simulink model "pole_placement_oldversion"  (R2022a)
settings: Solver=FixedStepAuto  StartTime=0.0  StopTime=10  FixedStep=0.001  RelTol=1e-3
values from neighbouring files (symbols this model uses):
  A = [0 1.51506314161 0 -114.917471751 0 1 -372.885867158 0 797.381461885 0 0 0.563745877458 ... (25 elements, 5x5)]    [System.mat]    (also in linearize_operating_point.m = double(A))
  B = [0 0 0 0 863.333333333]    [System.mat]    (also in linearize_operating_point.m = double(B))
  C = [1  0  0  0  0; 0  0  1  0  0]    [System.mat]    (also in linearize_operating_point.m = [1 0 0 0 0)
  D = [0 0]    [System.mat]    (also in linearize_operating_point.m = zeros(2,1))
  K = K1    [controller.m]
  Ke = place(A_, B_, 2*J)'    [controller.m]
  T_0 = x_op(5)    [controller.m]    (also in run_compare_lin_non_lin.m)
  theta_1_0 = x_op(1)    [controller.m]    (also in run_compare_lin_non_lin.m)
  theta_2_0 = x_op(3)    [controller.m]    (also in run_compare_lin_non_lin.m)
  theta_d_1_0 = x_op(2)    [controller.m]    (also in run_compare_lin_non_lin.m)
  theta_d_2_0 = x_op(4)    [controller.m]    (also in run_compare_lin_non_lin.m)
  x_op = [3.14159265359 0 0 0 0]    [System.mat]    (also in linearize_operating_point.m = [init_theta_1; 0; init_theta_2; 0; 0])
  x_op_relative = [0; 0; 0; 0; 0]    [controller.m]
libraries: slpidlib x4
(part 1 of 3)
settings Model: Creator=annel  LastModifiedBy=97083
settings ModelReferenceCC: EnableRefExpFcnMdlSchedulingChecks=off
settings RTWCC: Description=Generic Real-Time Target

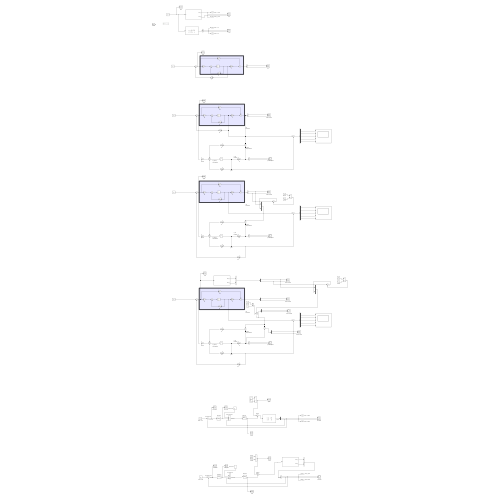
[thumbnail: Simulink's stored preview of the top-level diagram]
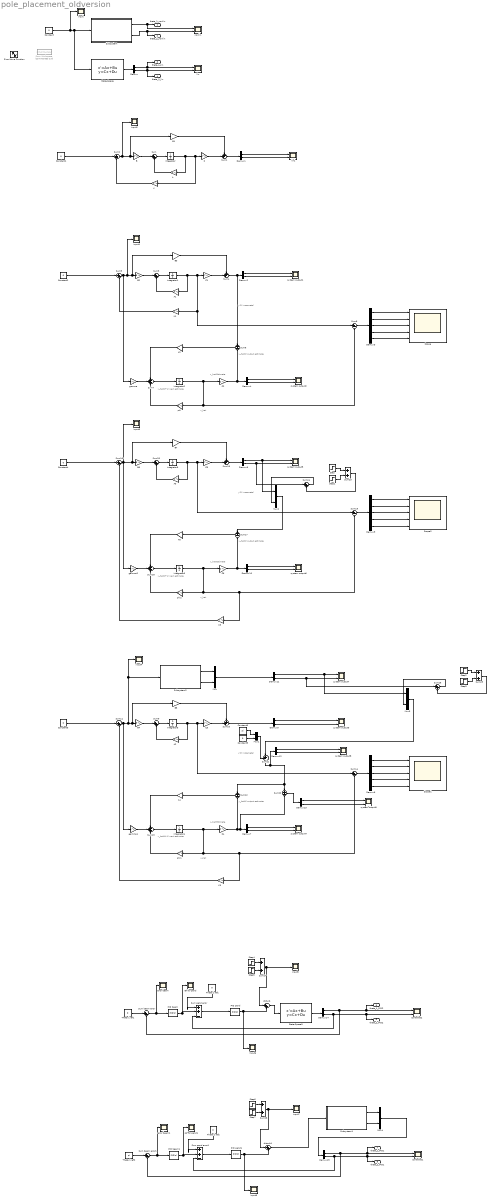
== system pole_placement_oldversion ==
  note: y_hat(k)
      | output estimate
  note: x_hat
  note: y(k)
      | incremetal
  note: x_hat(k+1)
      | next estimate
  note: x_hat
      | Estimate
  note: y_hat(k)
      | output estimate
  note: x_hat
  note: y(k)
      | incremetal
  note: x_hat(k+1)
      | next estimate
  note: x_hat
      | Estimate
  note: y_hat(k)
      | output estimate
  note: x_hat
  note: y(k)
      | incremetal
  note: x_hat(k+1)
      | next estimate
  note: x_hat
      | Estimate
  A{,1..3} (4 alike) : Gain  Gain=A  Multiplication=Matrix(K*u) (u vector)
  B{,2,4,6} (4 alike) : Gain  Gain=B  Multiplication=Matrix(K*u)
  B{1,3,5,7} (4 alike) : Gain  Gain=D  Multiplication=Matrix(K*u)
  C{,1..6} (7 alike) : Gain  Gain=C  Multiplication=Matrix(K*u) (u vector)
  Constant{,1..4} (5 alike) : Constant  Value=0  SampleTime=0.001
  Constant5 : Constant  Value=0  SampleTime=-1
  Constant6 : Constant  Value=pi  SampleTime=-1
  Demux{,1..2,4..5,7..8,10..15} (13 alike) : Demux  Outputs=2
  Demux3 : Demux  Outputs=5
  Demux6 : Demux  Outputs=5
  Demux9 : Demux  Outputs=5
  From Workspace : FromWorkspace  Commented=on  SampleTime=-1
  Integrator{,1..6} (7 alike) : Integrator  InitialCondition=x_op_relative
  K{,1,3,5} (4 alike) : Gain  Gain=K  Multiplication=Matrix(K*u) (u vector)
  K2 : Gain  Gain=Ke  Multiplication=Matrix(K*u) (u vector)
  K4 : Gain  Gain=Ke  Multiplication=Matrix(K*u) (u vector)
  K6 : Gain  Gain=Ke  Multiplication=Matrix(K*u) (u vector)
  Mux{,1..4} (5 alike) : Mux  Inputs=2
  PID beam : slpidlib/PID Controller  Controller=PID  Form=Parallel  TimeDomain=Continuous-time  UseExternalTs=off  SampleTime=-1  IntegratorMethod=Forward Euler  FilterMethod=Forward Euler  ControllerParametersSource=internal  P=-0.5  I=0  UseKiTs=off  D=-0.02  N=100  UseFilter=on  TunerSelectOption=Transfer Function Based (PID Tuner App)  InitialConditionSource=internal  InitialConditionForIntegrator=0  InitialConditionForFilter=0  DifferentiatorICPrevScaledInput=0  ExternalReset=none  TrackingMode=off  Kt=1  LimitOutput=off  SatLimitsSource=internal  UpperSaturationLimit=inf  LowerSaturationLimit=-inf  LinearizeAsGain=on  AntiWindupMode=none  Kb=1  POutMin=[]  POutMax=[]  IOutMin=[]  IOutMax=[]  DOutMin=[]  DOutMax=[]  NOutMin=[]  NOutMax=[]  SumOutMin=[]  SumOutMax=[]  SaturationOutMin=[]  SaturationOutMax=[]  PParamMin=[]  PParamMax=[]  IParamMin=[]  IParamMax=[]  DParamMin=[]  DParamMax=[]  NParamMin=[]  NParamMax=[]  KbParamMin=[]  KbParamMax=[]  KtParamMin=[]  KtParamMax=[]  KbOutMin=[]  KbOutMax=[]  KtOutMin=[]  KtOutMax=[]  IntegratorOutMin=[]  IntegratorOutMax=[]  FilterOutMin=[]  FilterOutMax=[]  SumI1OutMin=[]  SumI1OutMax=[]  SumI2OutMin=[]  SumI2OutMax=[]  SumI3OutMin=[]  SumI3OutMax=[]  SumI4OutMin=[]  SumI4OutMax=[]  SumDOutMin=[]  SumDOutMax=[]  DifferentiatorOutMin=[]  DifferentiatorOutMax=[]  FilterDiffOutCoefMin=[]  FilterDiffOutCoefMax=[]  ReciprocalOutMin=[]  ReciprocalOutMax=[]  SumDenOutMin=[]  SumDenOutMax=[]  SumNumOutMin=[]  SumNumOutMax=[]  DivideOutMin=[]  DivideOutMax=[]  UdiffTsProdOutMin=[]  UdiffTsProdOutMax=[]  NTsProdOutMin=[]  NTsProdOutMax=[]  UintegralTsProdOutMin=[]  UintegralTsProdOutMax=[]  UngainTsProdOutMin=[]  UngainTsProdOutMax=[]  IntegratorContinuousStateAttributes=''  IntegratorStateMustResolveToSignalObject=off  IntegratorRTWStateStorageClass=Auto  FilterContinuousStateAttributes=''  FilterStateMustResolveToSignalObject=off  FilterRTWStateStorageClass=Auto  ParallelPVariant=InternalParameters  IdealPVariant=Disabled  IVariant=InternalParameters  DVariant=InternalParameters  IntegratorVariant=Continuous  SatVariant=Disabled  AWVariant=Passthrough  PCopyVariant=Disabled  TRVariant=Disabled  FdbkBlocksVariant=Forward  IdealPFdbkVariant=Disabled  SatFdbkVariant=Disabled  DerivativeFilterVariant=ContFilter  NVariant=InternalParameters  NCopyVariant=Disabled  FilterICVariant=InternalICsFilter  IntegratorICVariant=InternalICs  ExternalResetVariant=Disabled  TRSumVariant=Passthrough  SumFdbkVariant=Disabled  SumVariant=Sum_PID  TsampFilterVariant=InternalTs  TsampNgainVariant=Passthrough  TsampIntegralVariant=Passthrough  ExternalSaturationOutDataTypeStr=Inherit: Same as second input
  PID beam1 : slpidlib/PID Controller  Controller=PID  Form=Parallel  TimeDomain=Continuous-time  UseExternalTs=off  SampleTime=-1  IntegratorMethod=Forward Euler  FilterMethod=Forward Euler  ControllerParametersSource=internal  P=-0.5  I=0  UseKiTs=off  D=-0.02  N=100  UseFilter=on  TunerSelectOption=Transfer Function Based (PID Tuner App)  InitialConditionSource=internal  InitialConditionForIntegrator=0  InitialConditionForFilter=0  DifferentiatorICPrevScaledInput=0  ExternalReset=none  TrackingMode=off  Kt=1  LimitOutput=off  SatLimitsSource=internal  UpperSaturationLimit=inf  LowerSaturationLimit=-inf  LinearizeAsGain=on  AntiWindupMode=none  Kb=1  POutMin=[]  POutMax=[]  IOutMin=[]  IOutMax=[]  DOutMin=[]  DOutMax=[]  NOutMin=[]  NOutMax=[]  SumOutMin=[]  SumOutMax=[]  SaturationOutMin=[]  SaturationOutMax=[]  PParamMin=[]  PParamMax=[]  IParamMin=[]  IParamMax=[]  DParamMin=[]  DParamMax=[]  NParamMin=[]  NParamMax=[]  KbParamMin=[]  KbParamMax=[]  KtParamMin=[]  KtParamMax=[]  KbOutMin=[]  KbOutMax=[]  KtOutMin=[]  KtOutMax=[]  IntegratorOutMin=[]  IntegratorOutMax=[]  FilterOutMin=[]  FilterOutMax=[]  SumI1OutMin=[]  SumI1OutMax=[]  SumI2OutMin=[]  SumI2OutMax=[]  SumI3OutMin=[]  SumI3OutMax=[]  SumI4OutMin=[]  SumI4OutMax=[]  SumDOutMin=[]  SumDOutMax=[]  DifferentiatorOutMin=[]  DifferentiatorOutMax=[]  FilterDiffOutCoefMin=[]  FilterDiffOutCoefMax=[]  ReciprocalOutMin=[]  ReciprocalOutMax=[]  SumDenOutMin=[]  SumDenOutMax=[]  SumNumOutMin=[]  SumNumOutMax=[]  DivideOutMin=[]  DivideOutMax=[]  UdiffTsProdOutMin=[]  UdiffTsProdOutMax=[]  NTsProdOutMin=[]  NTsProdOutMax=[]  UintegralTsProdOutMin=[]  UintegralTsProdOutMax=[]  UngainTsProdOutMin=[]  UngainTsProdOutMax=[]  IntegratorContinuousStateAttributes=''  IntegratorStateMustResolveToSignalObject=off  IntegratorRTWStateStorageClass=Auto  FilterContinuousStateAttributes=''  FilterStateMustResolveToSignalObject=off  FilterRTWStateStorageClass=Auto  ParallelPVariant=InternalParameters  IdealPVariant=Disabled  IVariant=InternalParameters  DVariant=InternalParameters  IntegratorVariant=Continuous  SatVariant=Disabled  AWVariant=Passthrough  PCopyVariant=Disabled  TRVariant=Disabled  FdbkBlocksVariant=Forward  IdealPFdbkVariant=Disabled  SatFdbkVariant=Disabled  DerivativeFilterVariant=ContFilter  NVariant=InternalParameters  NCopyVariant=Disabled  FilterICVariant=InternalICsFilter  IntegratorICVariant=InternalICs  ExternalResetVariant=Disabled  TRSumVariant=Passthrough  SumFdbkVariant=Disabled  SumVariant=Sum_PID  TsampFilterVariant=InternalTs  TsampNgainVariant=Passthrough  TsampIntegralVariant=Passthrough  ExternalSaturationOutDataTypeStr=Inherit: Same as second input
  PID pend : slpidlib/PID Controller  Controller=PID  Form=Parallel  TimeDomain=Continuous-time  UseExternalTs=off  SampleTime=-1  IntegratorMethod=Forward Euler  FilterMethod=Forward Euler  ControllerParametersSource=internal  P=-10  I=0  UseKiTs=off  D=-0.1  N=100  UseFilter=on  TunerSelectOption=Transfer Function Based (PID Tuner App)  InitialConditionSource=internal  InitialConditionForIntegrator=0  InitialConditionForFilter=0  DifferentiatorICPrevScaledInput=0  ExternalReset=none  TrackingMode=off  Kt=1  LimitOutput=off  SatLimitsSource=internal  UpperSaturationLimit=inf  LowerSaturationLimit=-inf  LinearizeAsGain=on  AntiWindupMode=none  Kb=1  POutMin=[]  POutMax=[]  IOutMin=[]  IOutMax=[]  DOutMin=[]  DOutMax=[]  NOutMin=[]  NOutMax=[]  SumOutMin=[]  SumOutMax=[]  SaturationOutMin=[]  SaturationOutMax=[]  PParamMin=[]  PParamMax=[]  IParamMin=[]  IParamMax=[]  DParamMin=[]  DParamMax=[]  NParamMin=[]  NParamMax=[]  KbParamMin=[]  KbParamMax=[]  KtParamMin=[]  KtParamMax=[]  KbOutMin=[]  KbOutMax=[]  KtOutMin=[]  KtOutMax=[]  IntegratorOutMin=[]  IntegratorOutMax=[]  FilterOutMin=[]  FilterOutMax=[]  SumI1OutMin=[]  SumI1OutMax=[]  SumI2OutMin=[]  SumI2OutMax=[]  SumI3OutMin=[]  SumI3OutMax=[]  SumI4OutMin=[]  SumI4OutMax=[]  SumDOutMin=[]  SumDOutMax=[]  DifferentiatorOutMin=[]  DifferentiatorOutMax=[]  FilterDiffOutCoefMin=[]  FilterDiffOutCoefMax=[]  ReciprocalOutMin=[]  ReciprocalOutMax=[]  SumDenOutMin=[]  SumDenOutMax=[]  SumNumOutMin=[]  SumNumOutMax=[]  DivideOutMin=[]  DivideOutMax=[]  UdiffTsProdOutMin=[]  UdiffTsProdOutMax=[]  NTsProdOutMin=[]  NTsProdOutMax=[]  UintegralTsProdOutMin=[]  UintegralTsProdOutMax=[]  UngainTsProdOutMin=[]  UngainTsProdOutMax=[]  IntegratorContinuousStateAttributes=''  IntegratorStateMustResolveToSignalObject=off  IntegratorRTWStateStorageClass=Auto  FilterContinuousStateAttributes=''  FilterStateMustResolveToSignalObject=off  FilterRTWStateStorageClass=Auto  ParallelPVariant=InternalParameters  IdealPVariant=Disabled  IVariant=InternalParameters  DVariant=InternalParameters  IntegratorVariant=Continuous  SatVariant=Disabled  AWVariant=Passthrough  PCopyVariant=Disabled  TRVariant=Disabled  FdbkBlocksVariant=Forward  IdealPFdbkVariant=Disabled  SatFdbkVariant=Disabled  DerivativeFilterVariant=ContFilter  NVariant=InternalParameters  NCopyVariant=Disabled  FilterICVariant=InternalICsFilter  IntegratorICVariant=InternalICs  ExternalResetVariant=Disabled  TRSumVariant=Passthrough  SumFdbkVariant=Disabled  SumVariant=Sum_PID  TsampFilterVariant=InternalTs  TsampNgainVariant=Passthrough  TsampIntegralVariant=Passthrough  ExternalSaturationOutDataTypeStr=Inherit: Same as second input
  PID pend1 : slpidlib/PID Controller  Controller=PID  Form=Parallel  TimeDomain=Continuous-time  UseExternalTs=off  SampleTime=-1  IntegratorMethod=Forward Euler  FilterMethod=Forward Euler  ControllerParametersSource=internal  P=-10  I=0  UseKiTs=off  D=-0.01  N=100  UseFilter=on  TunerSelectOption=Transfer Function Based (PID Tuner App)  InitialConditionSource=internal  InitialConditionForIntegrator=0  InitialConditionForFilter=0  DifferentiatorICPrevScaledInput=0  ExternalReset=none  TrackingMode=off  Kt=1  LimitOutput=off  SatLimitsSource=internal  UpperSaturationLimit=inf  LowerSaturationLimit=-inf  LinearizeAsGain=on  AntiWindupMode=none  Kb=1  POutMin=[]  POutMax=[]  IOutMin=[]  IOutMax=[]  DOutMin=[]  DOutMax=[]  NOutMin=[]  NOutMax=[]  SumOutMin=[]  SumOutMax=[]  SaturationOutMin=[]  SaturationOutMax=[]  PParamMin=[]  PParamMax=[]  IParamMin=[]  IParamMax=[]  DParamMin=[]  DParamMax=[]  NParamMin=[]  NParamMax=[]  KbParamMin=[]  KbParamMax=[]  KtParamMin=[]  KtParamMax=[]  KbOutMin=[]  KbOutMax=[]  KtOutMin=[]  KtOutMax=[]  IntegratorOutMin=[]  IntegratorOutMax=[]  FilterOutMin=[]  FilterOutMax=[]  SumI1OutMin=[]  SumI1OutMax=[]  SumI2OutMin=[]  SumI2OutMax=[]  SumI3OutMin=[]  SumI3OutMax=[]  SumI4OutMin=[]  SumI4OutMax=[]  SumDOutMin=[]  SumDOutMax=[]  DifferentiatorOutMin=[]  DifferentiatorOutMax=[]  FilterDiffOutCoefMin=[]  FilterDiffOutCoefMax=[]  ReciprocalOutMin=[]  ReciprocalOutMax=[]  SumDenOutMin=[]  SumDenOutMax=[]  SumNumOutMin=[]  SumNumOutMax=[]  DivideOutMin=[]  DivideOutMax=[]  UdiffTsProdOutMin=[]  UdiffTsProdOutMax=[]  NTsProdOutMin=[]  NTsProdOutMax=[]  UintegralTsProdOutMin=[]  UintegralTsProdOutMax=[]  UngainTsProdOutMin=[]  UngainTsProdOutMax=[]  IntegratorContinuousStateAttributes=''  IntegratorStateMustResolveToSignalObject=off  IntegratorRTWStateStorageClass=Auto  FilterContinuousStateAttributes=''  FilterStateMustResolveToSignalObject=off  FilterRTWStateStorageClass=Auto  ParallelPVariant=InternalParameters  IdealPVariant=Disabled  IVariant=InternalParameters  DVariant=InternalParameters  IntegratorVariant=Continuous  SatVariant=Disabled  AWVariant=Passthrough  PCopyVariant=Disabled  TRVariant=Disabled  FdbkBlocksVariant=Forward  IdealPFdbkVariant=Disabled  SatFdbkVariant=Disabled  DerivativeFilterVariant=ContFilter  NVariant=InternalParameters  NCopyVariant=Disabled  FilterICVariant=InternalICsFilter  IntegratorICVariant=InternalICs  ExternalResetVariant=Disabled  TRSumVariant=Passthrough  SumFdbkVariant=Disabled  SumVariant=Sum_PID  TsampFilterVariant=InternalTs  TsampNgainVariant=Passthrough  TsampIntegralVariant=Passthrough  ExternalSaturationOutDataTypeStr=Inherit: Same as second input
  Scope : Scope  NumInputPorts=5
  Scope1 : Scope  NumInputPorts=5
  Scope2 : Scope  NumInputPorts=5
  Sine Wave Function : Sin  Amplitude=0.1  Frequency=2*pi*2  SampleTime=0.001
  State-Space : StateSpace  A=A  B=B  C=C  D=D  InitialCondition=x_op
  State-Space3 : StateSpace  A=A  B=B  C=C  D=D  InitialCondition=x_op_relative
  Step : Step  After=0.2  SampleTime=0
  Step1 : Step  Time=1.05  After=-0.2  SampleTime=0
  Step2 : Step  After=2  SampleTime=0
  Step3 : Step  Time=1.05  After=-2  SampleTime=0
  Step4 : Step
  Step5 : Step  Time=1.1  After=-1
  Step6 : Step  After=2
  Step7 : Step  Time=1.05  After=-2
  Subsystem : Subsystem
  Subsystem1 : Subsystem
  Subsystem2 : Subsystem
  Sum{,3,9,20,24,26} (6 alike) : Sum  Inputs=|++
  Sum beam error : Sum  Inputs=|+-
  Sum beam error1 : Sum  Inputs=|+-
  Sum pend error : Sum  Inputs=|++-
  Sum pend error1 : Sum  Inputs=|++-
  Sum{1,4,10,15} (4 alike) : Sum  Inputs=++|
  Sum{2,5,8,11,14,16,19} (7 alike) : Sum  Inputs=|+-
  Sum{6,12,17,22} (4 alike) : Sum  Inputs=+|-
  Sum13 : Sum  Inputs=+++
  Sum18 : Sum  Inputs=+++
  Sum21 : Sum  Inputs=-+|
  Sum{23,25,27..28} (4 alike) : Sum
  Sum7 : Sum  Inputs=+++
  Theta 1 ref1 : Constant  Value=0
  Theta 1 ref2 : Constant  Value=pi
  Theta 2 ref1 : Constant  Value=0
  Theta 2 ref2 : Constant  Value=0
  controled1 : Scope  NumInputPorts=2
  controled2 : Scope  NumInputPorts=2
  disturb : Sum  Inputs=|++
  disturb1 : Sum  Inputs=|++
  error beam : Scope
  error beam1 : Scope
  gamma : Gain  Gain=B  Multiplication=Matrix(K*u)
  gamma1 : Gain  Gain=B  Multiplication=Matrix(K*u)
  gamma2 : Gain  Gain=B  Multiplication=Matrix(K*u)
  input{,1..8} (9 alike) : Scope
  lin : Scope  NumInputPorts=2
  lin1 : Scope  NumInputPorts=2
  nonlin : Scope  NumInputPorts=2
  phi : Gain  Gain=A  Multiplication=Matrix(K*u) (u vector)
  phi1 : Gain  Gain=A  Multiplication=Matrix(K*u) (u vector)
  phi2 : Gain  Gain=A  Multiplication=Matrix(K*u) (u vector)
  ref for pend : Scope
  ref for pend1 : Scope
  system output{1..9} (9 alike) : Scope  NumInputPorts=2
  theta_1_nonlin : Outport
  theta_2_nonlin : Outport  Port=2
  theta_1_lin : Outport  Port=3
  theta_2_lin : Outport  Port=4
  theta_1_PID2 : Outport  Port=5
  theta_2_PID2 : Outport  Port=6
  theta_1_PID1 : Outport  Port=7
  theta_2_PID1 : Outport  Port=8
  wires:
  Subsystem/1(theta_1) -> theta_1_nonlin/1, nonlin/1
  Constant/1 -> input/1, Subsystem/1(u), State-Space/1
  Subsystem/2(theta_2) -> theta_2_nonlin/1, nonlin/2
  Demux/1 -> theta_1_lin/1, lin/1
  Demux/2 -> theta_2_lin/1, lin/2
  State-Space/1 -> Demux/1
  B/1 -> Sum/1
  Sum/1 -> Integrator/1
  A/1 -> Sum/2
  C/1 -> Sum1/2
  Sum2/1 -> input2/1, B1/1, B/1  "u"
  Integrator/1 -> A/1, K/1, C/1
  Constant1/1 -> Sum2/1
  K/1 -> Sum2/2
  Sum1/1 -> Demux1/1
  Demux1/2 -> lin1/2
  Demux1/1 -> lin1/1
  B1/1 -> Sum1/1
  B3/1 -> Sum4/1
  Integrator1/1 -> A1/1, K1/1, Sum8/1, C1/1
  Demux2/1 -> system output1/1
  Demux2/2 -> system output1/2
  K1/1 -> Sum5/2
  C1/1 -> Sum4/2
  Constant2/1 -> Sum5/1
  Sum3/1 -> Integrator1/1
  Sum5/1 -> gamma/1, input1/1, B3/1, B2/1  "u"
  B2/1 -> Sum3/1
  A1/1 -> Sum3/2
  Integrator2/1 -> C2/1, Sum8/2, phi/1
  gamma/1 -> Sum7/2
  K2/1 -> Sum7/1
  Sum7/1 -> Integrator2/1
  Sum6/1 -> K2/1
  Sum4/1 -> Demux2/1, Sum6/1
  phi/1 -> Sum7/3
  Sum8/1 -> Demux3/1  "u"
  C2/1 -> Demux4/1, Sum6/2
  Demux4/2 -> system output2/2
  Demux4/1 -> system output2/1
  Demux3/1 -> Scope/1
  Demux3/2 -> Scope/2
  Demux3/3 -> Scope/3
  Demux3/4 -> Scope/4
  Demux3/5 -> Scope/5
  Demux6/5 -> Scope1/5
  Demux6/4 -> Scope1/4
  Demux6/3 -> Scope1/3
  Demux6/2 -> Scope1/2
  Demux6/1 -> Scope1/1
  Demux7/1 -> system output4/1
  Demux7/2 -> system output4/2
  C4/1 -> Sum12/2, Sum22/2, Demux7/1
  Sum14/1 -> Demux6/1  "u"
  phi1/1 -> Sum13/3
  Sum10/1 -> Demux5/1
  Sum12/1 -> K4/1
  Sum13/1 -> Integrator4/1
  K4/1 -> Sum13/1
  gamma1/1 -> Sum13/2
  Integrator4/1 -> phi1/1, K3/1, Sum14/2, C4/1
  A2/1 -> Sum9/2
  B4/1 -> Sum9/1
  Sum11/1 -> Subsystem2/1(u), input4/1, B4/1, B5/1, gamma1/1  "u"
  Sum9/1 -> Integrator3/1
  Constant3/1 -> Sum11/1
  C3/1 -> Sum10/2
  K3/1 -> Sum11/2
  Demux5/2 -> system output3/2
  Demux5/1 -> system output3/1
  Integrator3/1 -> C3/1, Sum14/1, A2/1
  B5/1 -> Sum10/1
  B7/1 -> Sum15/1
  Integrator5/1 -> A3/1, Sum19/1, C5/1
  Demux8/1 -> Mux2/1, system output5/1
  Demux8/2 -> Sum24/1, system output5/2
  K5/1 -> Sum16/2
  C5/1 -> Sum15/2
  Constant4/1 -> Sum16/1
  Sum20/1 -> Integrator5/1
  Sum16/1 -> input3/1, gamma2/1, B7/1, B6/1  "u"
  B6/1 -> Sum20/1
  A3/1 -> Sum20/2
  Integrator6/1 -> C6/1, Sum19/2, K5/1, phi2/1
  gamma2/1 -> Sum18/2
  K6/1 -> Sum18/1
  Sum18/1 -> Integrator6/1
  Sum17/1 -> K6/1
  Sum15/1 -> Demux8/1
  phi2/1 -> Sum18/3
  Sum19/1 -> Demux9/1  "u"
  C6/1 -> Demux10/1, Sum17/2
  Demux10/2 -> system output6/2
  Demux10/1 -> system output6/1
  Demux9/1 -> Scope2/1
  Demux9/2 -> Scope2/2
  Demux9/3 -> Scope2/3
  Demux9/4 -> Scope2/4
  Demux9/5 -> Scope2/5
  Subsystem2/1(theta_1) -> Mux/1
  Subsystem2/2(theta_2) -> Mux/2
  Mux/1 -> Demux11/1
  Constant6/1 -> Mux1/1
  Constant5/1 -> Mux1/2
  Mux1/1 -> Sum21/1
  Sum21/1 -> Sum12/1, Sum22/1, Demux12/1
  Demux12/1 -> system output8/1
  Demux12/2 -> system output8/2
  Sum22/1 -> Demux13/1
  Demux13/2 -> system output9/2
  Demux13/1 -> system output9/1
  Mux2/1 -> Sum17/1
  Step/1 -> Sum23/1
  Step1/1 -> Sum23/2
  Sum23/1 -> Sum24/2  "u"
  Sum24/1 -> Mux2/2  "u"
  Demux11/2 -> Sum26/1, system output7/2
  Sum26/1 -> Mux3/2  "u"
  Sum25/1 -> Sum26/2  "u"
  Step2/1 -> Sum25/1
  Demux11/1 -> Mux3/1, system output7/1
  Step3/1 -> Sum25/2
  Mux3/1 -> Sum21/2
  Sum27/1 -> input5/1, disturb/1
  Step5/1 -> Sum27/2
  disturb/1 -> State-Space3/1  "error term"
  Theta 2 ref1/1 -> Sum pend error/1
  PID pend/1 -> input6/1, disturb/2
  Step4/1 -> Sum27/1
  State-Space3/1 -> Demux14/1  "output y"
  Demux14/2 -> Sum pend error/3, theta_2_PID2/1, controled2/2
  Demux14/1 -> theta_1_PID2/1, controled2/1, Sum beam error/2
  Sum pend error/1 -> PID pend/1  "error term"
  Sum beam error/1 -> error beam/1, PID beam/1  "error term"
  PID beam/1 -> ref for pend/1, Sum pend error/2
  Theta 1 ref1/1 -> Sum beam error/1
  Theta 1 ref2/1 -> Sum beam error1/1
  PID beam1/1 -> ref for pend1/1, Sum pend error1/2
  Mux4/1 -> Demux15/1  "output y"
  Step6/1 -> Sum28/1
  Sum pend error1/1 -> PID pend1/1  "error term"
  Demux15/2 -> Sum pend error1/3, theta_2_PID1/1, controled1/2
  Demux15/1 -> theta_1_PID1/1, controled1/1, Sum beam error1/2
  PID pend1/1 -> input8/1, disturb1/2
  Step7/1 -> Sum28/2
  Sum28/1 -> input7/1, disturb1/1
  Theta 2 ref2/1 -> Sum pend error1/1
  Sum beam error1/1 -> error beam1/1, PID beam1/1  "error term"
  disturb1/1 -> Subsystem1/1(u)  "u"
  Subsystem1/1(theta_1) -> Mux4/1
  Subsystem1/2(theta_2) -> Mux4/2

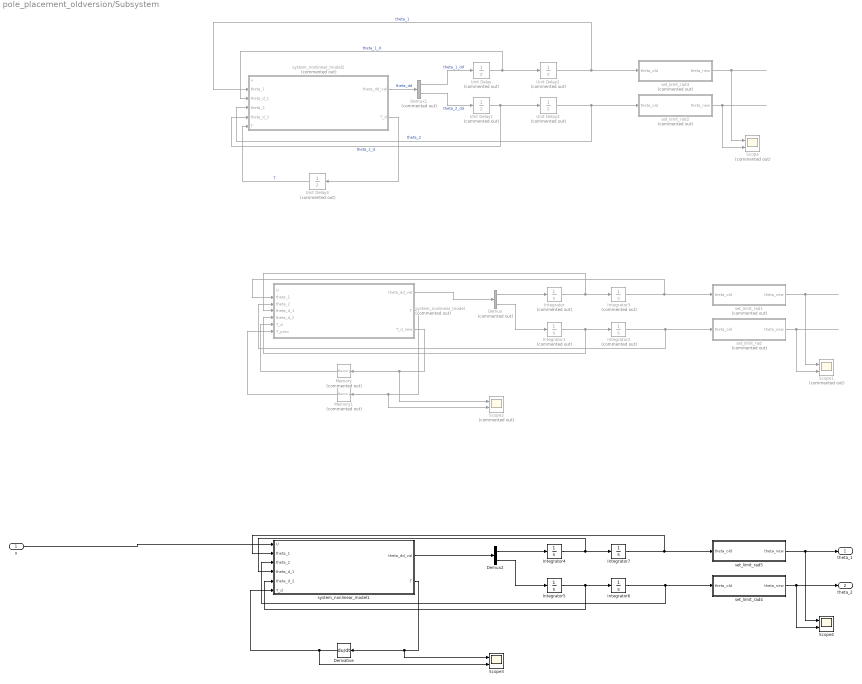
== system pole_placement_oldversion/Subsystem ==
  u : Inport
  Demux : Demux  Commented=on  Outputs=2
  Demux1 : Demux  Commented=on  Outputs=2
  Demux2 : Demux  Outputs=2
  Derivative : Derivative
  Integrator : Integrator  Commented=on
  Integrator1 : Integrator  Commented=on
  Integrator2 : Integrator  Commented=on  InitialCondition=theta_2_0
  Integrator3 : Integrator  Commented=on  InitialCondition=theta_1_0
  Integrator4 : Integrator
  Integrator5 : Integrator
  Integrator6 : Integrator  InitialCondition=theta_2_0
  Integrator7 : Integrator  InitialCondition=theta_1_0
  Memory : Memory  Commented=on  InheritSampleTime=on
  Memory1 : Memory  Commented=on  InheritSampleTime=on
  Scope : Scope  Commented=on  NumInputPorts=2
  Scope1 : Scope  Commented=on  NumInputPorts=2
  Scope2 : Scope  Commented=on  NumInputPorts=2
  Scope3 : Scope  NumInputPorts=2
  Scope4 : Scope  NumInputPorts=2
  Unit Delay : UnitDelay  Commented=on  InitialCondition=theta_d_1_0  SampleTime=-1  HasFrameUpgradeWarning=on
  Unit Delay1 : UnitDelay  Commented=on  InitialCondition=theta_d_2_0  SampleTime=-1  HasFrameUpgradeWarning=on
  Unit Delay2 : UnitDelay  Commented=on  InitialCondition=theta_1_0  SampleTime=-1  HasFrameUpgradeWarning=on
  Unit Delay3 : UnitDelay  Commented=on  InitialCondition=theta_2_0  SampleTime=-1  HasFrameUpgradeWarning=on
  Unit Delay4 : UnitDelay  Commented=on  InitialCondition=T_0  SampleTime=-1  HasFrameUpgradeWarning=on
  set_limit_rad : MATLAB Function  Commented=on  TreatAsAtomicUnit=on
  set_limit_rad1 : MATLAB Function  Commented=on  TreatAsAtomicUnit=on
  set_limit_rad2 : MATLAB Function  Commented=on  TreatAsAtomicUnit=on
  set_limit_rad3 : MATLAB Function  Commented=on  TreatAsAtomicUnit=on
  set_limit_rad4 : MATLAB Function  TreatAsAtomicUnit=on
  set_limit_rad5 : MATLAB Function  TreatAsAtomicUnit=on
  system_nonlinear_model : MATLAB Function  Commented=on  TreatAsAtomicUnit=on
  system_nonlinear_model1 : MATLAB Function  TreatAsAtomicUnit=on
  system_nonlinear_model2 : MATLAB Function  Commented=on  TreatAsAtomicUnit=on
  theta_1 : Outport
  theta_2 : Outport  Port=2
  wires:
  set_limit_rad3/1(theta_new) -> Scope/1
  Unit Delay2/1 -> system_nonlinear_model2/2(theta_1), set_limit_rad3/1(theta_old)  "theta_1"
  Unit Delay3/1 -> system_nonlinear_model2/4(theta_2), set_limit_rad2/1(theta_old)  "theta_2"
  ? -> system_nonlinear_model2/1(u)
  Unit Delay1/1 -> system_nonlinear_model2/5(theta_d_2), Unit Delay3/1  "theta_2_d"
  set_limit_rad2/1(theta_new) -> Scope/2
  system_nonlinear_model2/1(theta_dd_val) -> Demux1/1  "theta_dd"
  Demux1/2 -> Unit Delay1/1  "theta_2_dd"
  Demux1/1 -> Unit Delay/1  "theta_1_dd"
  Unit Delay/1 -> system_nonlinear_model2/3(theta_d_1), Unit Delay2/1  "theta_1_d"
  system_nonlinear_model2/2(T_d) -> Unit Delay4/1
  Unit Delay4/1 -> system_nonlinear_model2/6(T)  "T"
  Memory/1 -> system_nonlinear_model/6(T_d)
  Memory1/1 -> system_nonlinear_model/7(T_prev)
  Integrator/1 -> system_nonlinear_model/4(theta_d_1), Integrator3/1
  system_nonlinear_model/3(T_d_new) -> Scope2/1, Memory/1
  Integrator1/1 -> system_nonlinear_model/5(theta_d_2), Integrator2/1
  ? -> system_nonlinear_model/1(U)
  Integrator2/1 -> system_nonlinear_model/3(theta_2), set_limit_rad/1(theta_old)
  Integrator3/1 -> set_limit_rad1/1(theta_old), system_nonlinear_model/2(theta_1)
  system_nonlinear_model/2(T) -> Scope2/2, Memory1/1
  set_limit_rad/1(theta_new) -> Scope1/2
  Demux/1 -> Integrator/1
  system_nonlinear_model/1(theta_dd_val) -> Demux/1
  Demux/2 -> Integrator1/1
  set_limit_rad1/1(theta_new) -> Scope1/1
  set_limit_rad5/1(theta_new) -> theta_1/1, Scope4/1
  Demux2/2 -> Integrator5/1
  Integrator6/1 -> system_nonlinear_model1/3(theta_2), set_limit_rad4/1(theta_old)
  Demux2/1 -> Integrator4/1
  system_nonlinear_model1/1(theta_dd_val) -> Demux2/1
  Integrator5/1 -> system_nonlinear_model1/5(theta_d_2), Integrator6/1
  Integrator7/1 -> set_limit_rad5/1(theta_old), system_nonlinear_model1/2(theta_1)
  system_nonlinear_model1/2(T) -> Scope3/1, Derivative/1
  set_limit_rad4/1(theta_new) -> theta_2/1, Scope4/2
  u/1 -> system_nonlinear_model1/1(U)
  Integrator4/1 -> system_nonlinear_model1/4(theta_d_1), Integrator7/1
  Derivative/1 -> Scope3/2, system_nonlinear_model1/6(T_d)

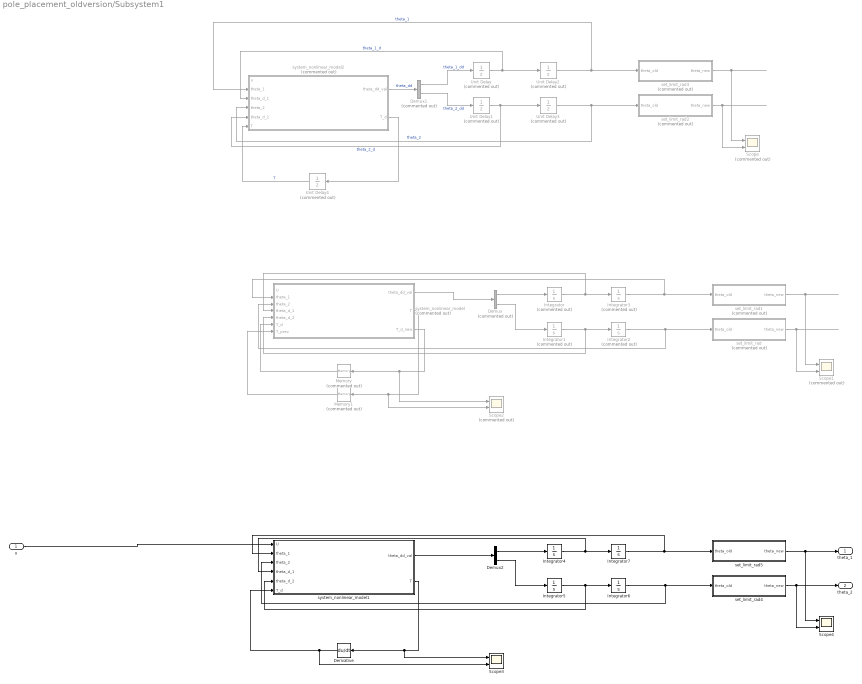
== system pole_placement_oldversion/Subsystem1 ==
  u : Inport
  Demux : Demux  Commented=on  Outputs=2
  Demux1 : Demux  Commented=on  Outputs=2
  Demux2 : Demux  Outputs=2
  Derivative : Derivative
  Integrator : Integrator  Commented=on
  Integrator1 : Integrator  Commented=on
  Integrator2 : Integrator  Commented=on  InitialCondition=theta_2_0
  Integrator3 : Integrator  Commented=on  InitialCondition=theta_1_0
  Integrator4 : Integrator
  Integrator5 : Integrator
  Integrator6 : Integrator  InitialCondition=theta_2_0
  Integrator7 : Integrator  InitialCondition=theta_1_0
  Memory : Memory  Commented=on  InheritSampleTime=on
  Memory1 : Memory  Commented=on  InheritSampleTime=on
  Scope : Scope  Commented=on  NumInputPorts=2
  Scope1 : Scope  Commented=on  NumInputPorts=2
  Scope2 : Scope  Commented=on  NumInputPorts=2
  Scope3 : Scope  NumInputPorts=2
  Scope4 : Scope  NumInputPorts=2
  Unit Delay : UnitDelay  Commented=on  InitialCondition=theta_d_1_0  SampleTime=-1  HasFrameUpgradeWarning=on
  Unit Delay1 : UnitDelay  Commented=on  InitialCondition=theta_d_2_0  SampleTime=-1  HasFrameUpgradeWarning=on
  Unit Delay2 : UnitDelay  Commented=on  InitialCondition=theta_1_0  SampleTime=-1  HasFrameUpgradeWarning=on
  Unit Delay3 : UnitDelay  Commented=on  InitialCondition=theta_2_0  SampleTime=-1  HasFrameUpgradeWarning=on
  Unit Delay4 : UnitDelay  Commented=on  InitialCondition=T_0  SampleTime=-1  HasFrameUpgradeWarning=on
  set_limit_rad : MATLAB Function  Commented=on  TreatAsAtomicUnit=on
  set_limit_rad1 : MATLAB Function  Commented=on  TreatAsAtomicUnit=on
  set_limit_rad2 : MATLAB Function  Commented=on  TreatAsAtomicUnit=on
  set_limit_rad3 : MATLAB Function  Commented=on  TreatAsAtomicUnit=on
  set_limit_rad4 : MATLAB Function  TreatAsAtomicUnit=on
  set_limit_rad5 : MATLAB Function  TreatAsAtomicUnit=on
  system_nonlinear_model : MATLAB Function  Commented=on  TreatAsAtomicUnit=on
  system_nonlinear_model1 : MATLAB Function  TreatAsAtomicUnit=on
  system_nonlinear_model2 : MATLAB Function  Commented=on  TreatAsAtomicUnit=on
  theta_1 : Outport
  theta_2 : Outport  Port=2
  wires:
  set_limit_rad3/1(theta_new) -> Scope/1
  Unit Delay2/1 -> system_nonlinear_model2/2(theta_1), set_limit_rad3/1(theta_old)  "theta_1"
  Unit Delay3/1 -> system_nonlinear_model2/4(theta_2), set_limit_rad2/1(theta_old)  "theta_2"
  ? -> system_nonlinear_model2/1(u)
  Unit Delay1/1 -> system_nonlinear_model2/5(theta_d_2), Unit Delay3/1  "theta_2_d"
  set_limit_rad2/1(theta_new) -> Scope/2
  system_nonlinear_model2/1(theta_dd_val) -> Demux1/1  "theta_dd"
  Demux1/2 -> Unit Delay1/1  "theta_2_dd"
  Demux1/1 -> Unit Delay/1  "theta_1_dd"
  Unit Delay/1 -> system_nonlinear_model2/3(theta_d_1), Unit Delay2/1  "theta_1_d"
  system_nonlinear_model2/2(T_d) -> Unit Delay4/1
  Unit Delay4/1 -> system_nonlinear_model2/6(T)  "T"
  Memory/1 -> system_nonlinear_model/6(T_d)
  Memory1/1 -> system_nonlinear_model/7(T_prev)
  Integrator/1 -> system_nonlinear_model/4(theta_d_1), Integrator3/1
  system_nonlinear_model/3(T_d_new) -> Scope2/1, Memory/1
  Integrator1/1 -> system_nonlinear_model/5(theta_d_2), Integrator2/1
  ? -> system_nonlinear_model/1(U)
  Integrator2/1 -> system_nonlinear_model/3(theta_2), set_limit_rad/1(theta_old)
  Integrator3/1 -> set_limit_rad1/1(theta_old), system_nonlinear_model/2(theta_1)
  system_nonlinear_model/2(T) -> Scope2/2, Memory1/1
  set_limit_rad/1(theta_new) -> Scope1/2
  Demux/1 -> Integrator/1
  system_nonlinear_model/1(theta_dd_val) -> Demux/1
  Demux/2 -> Integrator1/1
  set_limit_rad1/1(theta_new) -> Scope1/1
  set_limit_rad5/1(theta_new) -> theta_1/1, Scope4/1
  Demux2/2 -> Integrator5/1
  Integrator6/1 -> system_nonlinear_model1/3(theta_2), set_limit_rad4/1(theta_old)
  Demux2/1 -> Integrator4/1
  system_nonlinear_model1/1(theta_dd_val) -> Demux2/1
  Integrator5/1 -> system_nonlinear_model1/5(theta_d_2), Integrator6/1
  Integrator7/1 -> set_limit_rad5/1(theta_old), system_nonlinear_model1/2(theta_1)
  system_nonlinear_model1/2(T) -> Scope3/1, Derivative/1
  set_limit_rad4/1(theta_new) -> theta_2/1, Scope4/2
  u/1 -> system_nonlinear_model1/1(U)
  Integrator4/1 -> system_nonlinear_model1/4(theta_d_1), Integrator7/1
  Derivative/1 -> Scope3/2, system_nonlinear_model1/6(T_d)

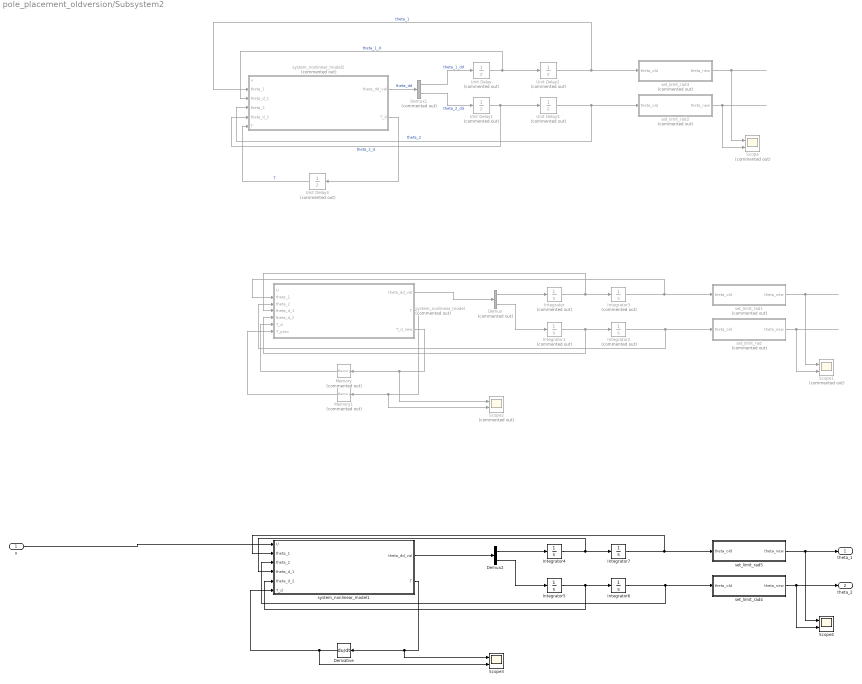
== system pole_placement_oldversion/Subsystem2 ==
  u : Inport
  Demux : Demux  Commented=on  Outputs=2
  Demux1 : Demux  Commented=on  Outputs=2
  Demux2 : Demux  Outputs=2
  Derivative : Derivative
  Integrator : Integrator  Commented=on
  Integrator1 : Integrator  Commented=on
  Integrator2 : Integrator  Commented=on  InitialCondition=theta_2_0
  Integrator3 : Integrator  Commented=on  InitialCondition=theta_1_0
  Integrator4 : Integrator
  Integrator5 : Integrator
  Integrator6 : Integrator  InitialCondition=theta_2_0
  Integrator7 : Integrator  InitialCondition=theta_1_0
  Memory : Memory  Commented=on  InheritSampleTime=on
  Memory1 : Memory  Commented=on  InheritSampleTime=on
  Scope : Scope  Commented=on  NumInputPorts=2
  Scope1 : Scope  Commented=on  NumInputPorts=2
  Scope2 : Scope  Commented=on  NumInputPorts=2
  Scope3 : Scope  NumInputPorts=2
  Scope4 : Scope  NumInputPorts=2
  Unit Delay : UnitDelay  Commented=on  InitialCondition=theta_d_1_0  SampleTime=-1  HasFrameUpgradeWarning=on
  Unit Delay1 : UnitDelay  Commented=on  InitialCondition=theta_d_2_0  SampleTime=-1  HasFrameUpgradeWarning=on
  Unit Delay2 : UnitDelay  Commented=on  InitialCondition=theta_1_0  SampleTime=-1  HasFrameUpgradeWarning=on
  Unit Delay3 : UnitDelay  Commented=on  InitialCondition=theta_2_0  SampleTime=-1  HasFrameUpgradeWarning=on
  Unit Delay4 : UnitDelay  Commented=on  InitialCondition=T_0  SampleTime=-1  HasFrameUpgradeWarning=on
  set_limit_rad : MATLAB Function  Commented=on  TreatAsAtomicUnit=on
  set_limit_rad1 : MATLAB Function  Commented=on  TreatAsAtomicUnit=on
  set_limit_rad2 : MATLAB Function  Commented=on  TreatAsAtomicUnit=on
  set_limit_rad3 : MATLAB Function  Commented=on  TreatAsAtomicUnit=on
  set_limit_rad4 : MATLAB Function  TreatAsAtomicUnit=on
  set_limit_rad5 : MATLAB Function  TreatAsAtomicUnit=on
  system_nonlinear_model : MATLAB Function  Commented=on  TreatAsAtomicUnit=on
  system_nonlinear_model1 : MATLAB Function  TreatAsAtomicUnit=on
  system_nonlinear_model2 : MATLAB Function  Commented=on  TreatAsAtomicUnit=on
  theta_1 : Outport
  theta_2 : Outport  Port=2
  wires:
  set_limit_rad3/1(theta_new) -> Scope/1
  Unit Delay2/1 -> system_nonlinear_model2/2(theta_1), set_limit_rad3/1(theta_old)  "theta_1"
  Unit Delay3/1 -> system_nonlinear_model2/4(theta_2), set_limit_rad2/1(theta_old)  "theta_2"
  ? -> system_nonlinear_model2/1(u)
  Unit Delay1/1 -> system_nonlinear_model2/5(theta_d_2), Unit Delay3/1  "theta_2_d"
  set_limit_rad2/1(theta_new) -> Scope/2
  system_nonlinear_model2/1(theta_dd_val) -> Demux1/1  "theta_dd"
  Demux1/2 -> Unit Delay1/1  "theta_2_dd"
  Demux1/1 -> Unit Delay/1  "theta_1_dd"
  Unit Delay/1 -> system_nonlinear_model2/3(theta_d_1), Unit Delay2/1  "theta_1_d"
  system_nonlinear_model2/2(T_d) -> Unit Delay4/1
  Unit Delay4/1 -> system_nonlinear_model2/6(T)  "T"
  Memory/1 -> system_nonlinear_model/6(T_d)
  Memory1/1 -> system_nonlinear_model/7(T_prev)
  Integrator/1 -> system_nonlinear_model/4(theta_d_1), Integrator3/1
  system_nonlinear_model/3(T_d_new) -> Scope2/1, Memory/1
  Integrator1/1 -> system_nonlinear_model/5(theta_d_2), Integrator2/1
  ? -> system_nonlinear_model/1(U)
  Integrator2/1 -> system_nonlinear_model/3(theta_2), set_limit_rad/1(theta_old)
  Integrator3/1 -> set_limit_rad1/1(theta_old), system_nonlinear_model/2(theta_1)
  system_nonlinear_model/2(T) -> Scope2/2, Memory1/1
  set_limit_rad/1(theta_new) -> Scope1/2
  Demux/1 -> Integrator/1
  system_nonlinear_model/1(theta_dd_val) -> Demux/1
  Demux/2 -> Integrator1/1
  set_limit_rad1/1(theta_new) -> Scope1/1
  set_limit_rad5/1(theta_new) -> theta_1/1, Scope4/1
  Demux2/2 -> Integrator5/1
  Integrator6/1 -> system_nonlinear_model1/3(theta_2), set_limit_rad4/1(theta_old)
  Demux2/1 -> Integrator4/1
  system_nonlinear_model1/1(theta_dd_val) -> Demux2/1
  Integrator5/1 -> system_nonlinear_model1/5(theta_d_2), Integrator6/1
  Integrator7/1 -> set_limit_rad5/1(theta_old), system_nonlinear_model1/2(theta_1)
  system_nonlinear_model1/2(T) -> Scope3/1, Derivative/1
  set_limit_rad4/1(theta_new) -> theta_2/1, Scope4/2
  u/1 -> system_nonlinear_model1/1(U)
  Integrator4/1 -> system_nonlinear_model1/4(theta_d_1), Integrator7/1
  Derivative/1 -> Scope3/2, system_nonlinear_model1/6(T_d)

== matlab function pole_placement_oldversion/Subsystem1/set_limit_rad2 ==
  settings: updateMethod=DISCRETE  sampleTime=0.001
  data: theta_old input size=1; theta_new output size=1
function theta_new   = set_limit_rad(theta_old)

theta_new = theta_old - floor(theta_old / 2 / pi) * 2 * pi;
theta_new = theta_old;

== matlab function pole_placement_oldversion/Subsystem1/set_limit_rad3 ==
  settings: updateMethod=DISCRETE  sampleTime=0.001
  data: theta_old input size=1; theta_new output size=1
function theta_new   = set_limit_rad(theta_old)

theta_new = theta_old - floor(theta_old / 2 / pi) * 2 * pi;
theta_new = theta_old;

== matlab function pole_placement_oldversion/Subsystem1/set_limit_rad4 ==
  settings: updateMethod=DISCRETE  sampleTime=0.001
  data: theta_old input size=1; theta_new output size=1
function theta_new   = set_limit_rad(theta_old)

theta_new = theta_old - floor(theta_old / 2 / pi) * 2 * pi;
theta_new = theta_old;

== matlab function pole_placement_oldversion/Subsystem1/set_limit_rad5 ==
  settings: updateMethod=DISCRETE  sampleTime=0.001
  data: theta_old input size=1; theta_new output size=1
function theta_new   = set_limit_rad(theta_old)

theta_new = theta_old - floor(theta_old / 2 / pi) * 2 * pi;
theta_new = theta_old;

== matlab function pole_placement_oldversion/Subsystem/set_limit_rad4 ==
  settings: updateMethod=DISCRETE  sampleTime=0.001
  data: theta_old input size=1; theta_new output size=1
function theta_new   = set_limit_rad(theta_old)

theta_new = theta_old - floor(theta_old / 2 / pi) * 2 * pi;
theta_new = theta_old;

== matlab function pole_placement_oldversion/Subsystem/set_limit_rad5 ==
  settings: updateMethod=DISCRETE  sampleTime=0.001
  data: theta_old input size=1; theta_new output size=1
function theta_new   = set_limit_rad(theta_old)

theta_new = theta_old - floor(theta_old / 2 / pi) * 2 * pi;
theta_new = theta_old;

== matlab function pole_placement_oldversion/Subsystem/system_nonlinear_model1 ==
  settings: updateMethod=DISCRETE  sampleTime=0.001
  data: U input size=1; theta_dd_val output size=2; T output; theta_1 input size=1; theta_2 input size=1; theta_d_1 input size=1; theta_d_2 input size=1; T_d input
function [theta_dd_val, T]   = get_theta_dt_dt(U, theta_1, theta_2, theta_d_1, theta_d_2, T_d)


u = U(1);
k_m_0 = 15;
tau_e_0 = 0.03;

T = k_m_0 * u - tau_e_0 * T_d;



% theta_dd_val = [
%                                                                                                                                                                    (2177205792337185200000*sin(theta_1 + theta_2)*(7101996468378179*cos(theta_2) + 5837472162125388))/(59390441777463697512*cos(theta_2) + 157619855740175396464645510487628125*cos(theta_2)^2 - 67469767625708245300871903596602750000) - theta_d_2*((1152921504606846976*(7101996468378179*cos(theta_2) + 5837472162125388))/(59390441777463697512*cos(theta_2) + 157619855740175396464645510487628125*cos(theta_2)^2 - 67469767625708245300871903596602750000) + (336507359412909324930676272031334400000*sin(theta_2)*((7101996468378179*theta_d_1)/18446744073709551616 + (7101996468378179*theta_d_2)/18446744073709551616))/(59390441777463697512*cos(theta_2) + 157619855740175396464645510487628125*cos(theta_2)^2 - 67469767625708245300871903596602750000)) - theta_d_1*((336507359412909324930676272031334400000*((7101996468378179*theta_d_2*sin(theta_2))/18446744073709551616 - 5171/250))/(59390441777463697512*cos(theta_2) + 157619855740175396464645510487628125*cos(theta_2)^2 - 67469767625708245300871903596602750000) + (22193738963681809375*theta_d_1*sin(theta_2)*(7101996468378179*cos(theta_2) + 5837472162125388))/(59390441777463697512*cos(theta_2) + 157619855740175396464645510487628125*cos(theta_2)^2 - 67469767625708245300871903596602750000)) - (336507359412909324930676272031334400000*T)/(59390441777463697512*cos(theta_2) + 157619855740175396464645510487628125*cos(theta_2)^2 - 67469767625708245300871903596602750000) - (336507359412909324930676272031334400000*((5443014480842963*sin(theta_1 + theta_2))/144115188075855872 + (3446064362871357*sin(theta_1))/72057594037927936))/(59390441777463697512*cos(theta_2) + 157619855740175396464645510487628125*cos(theta_2)^2 - 67469767625708245300871903596602750000);
% theta_d_1*((57646075230342348800000*(7101996468378179*cos(theta_2) + 5837472162125388)*((7101996468378179*theta_d_2*sin(theta_2))/18446744073709551616 - 5171/250))/(59390441777463697512*cos(theta_2) + 157619855740175396464645510487628125*cos(theta_2)^2 - 67469767625708245300871903596602750000) + (7272444383619255296*theta_d_1*sin(theta_2)*(43347146413441024*cos(theta_2) + 11304968154247740625))/(59390441777463697512*cos(theta_2) + 157619855740175396464645510487628125*cos(theta_2)^2 - 67469767625708245300871903596602750000)) + theta_d_2*((1180591620717411303424*(43347146413441024*cos(theta_2) + 11304968154247740625))/(3125*(59390441777463697512*cos(theta_2) + 157619855740175396464645510487628125*cos(theta_2)^2 - 67469767625708245300871903596602750000)) + (57646075230342348800000*sin(theta_2)*(7101996468378179*cos(theta_2) + 5837472162125388)*((7101996468378179*theta_d_1)/18446744073709551616 + (7101996468378179*theta_d_2)/18446744073709551616))/(59390441777463697512*cos(theta_2) + 157619855740175396464645510487628125*cos(theta_2)^2 - 67469767625708245300871903596602750000)) + (57646075230342348800000*T*(7101996468378179*cos(theta_2) + 5837472162125388))/(59390441777463697512*cos(theta_2) + 157619855740175396464645510487628125*cos(theta_2)^2 - 67469767625708245300871903596602750000) + (57646075230342348800000*(7101996468378179*cos(theta_2) + 5837472162125388)*((5443014480842963*sin(theta_1 + theta_2))/144115188075855872 + (3446064362871357*sin(theta_1))/72057594037927936))/(59390441777463697512*cos(theta_2) + 157619855740175396464645510487628125*cos(theta_2)^2 - 67469767625708245300871903596602750000) - (713426794033048846336*sin(theta_1 + theta_2)*(43347146413441024*cos(theta_2) + 11304968154247740625))/(59390441777463697512*cos(theta_2) + 157619855740175396464645510487628125*cos(theta_2)^2 - 67469767625708245300871903596602750000)];
%  
%                                                                                                        (50632000000*((3*T_d)/100 - 15*u))/(7*(3388000*cos(theta_2)^2 - 1450246047)) - theta_d_2*((160*(7700*cos(theta_2) + 6329))/(7*(3388000*cos(theta_2)^2 - 1450246047)) + (50632000000*sin(theta_2)*((77*theta_d_1)/200000 + (77*theta_d_2)/200000))/(7*(3388000*cos(theta_2)^2 - 1450246047))) - (50632000000*((75537*sin(theta_1 + theta_2))/2000000 + (38259*sin(theta_1))/800000))/(7*(3388000*cos(theta_2)^2 - 1450246047)) - theta_d_1*((50632000000*((77*theta_d_2*sin(theta_2))/200000 - 5171/250))/(7*(3388000*cos(theta_2)^2 - 1450246047)) + (440*theta_d_1*sin(theta_2)*(7700*cos(theta_2) + 6329))/(3388000*cos(theta_2)^2 - 1450246047)) + (43164*sin(theta_1 + theta_2)*(7700*cos(theta_2) + 6329))/(3388000*cos(theta_2)^2 - 1450246047);
% theta_d_2*((80*(30800*cos(theta_2) + 8032663))/(7*(3388000*cos(theta_2)^2 - 1450246047)) + (8000000*sin(theta_2)*((77*theta_d_1)/200000 + (77*theta_d_2)/200000)*(7700*cos(theta_2) + 6329))/(7*(3388000*cos(theta_2)^2 - 1450246047))) + theta_d_1*((8000000*((77*theta_d_2*sin(theta_2))/200000 - 5171/250)*(7700*cos(theta_2) + 6329))/(7*(3388000*cos(theta_2)^2 - 1450246047)) + (220*theta_d_1*sin(theta_2)*(30800*cos(theta_2) + 8032663))/(3388000*cos(theta_2)^2 - 1450246047)) - (21582*sin(theta_1 + theta_2)*(30800*cos(theta_2) + 8032663))/(3388000*cos(theta_2)^2 - 1450246047) + (8000000*(7700*cos(theta_2) + 6329)*((75537*sin(theta_1 + theta_2))/2000000 + (38259*sin(theta_1))/800000))/(7*(3388000*cos(theta_2)^2 - 1450246047)) - (8000000*(7700*cos(theta_2) + 6329)*((3*T_d)/100 - 15*u))/(7*(3388000*cos(theta_2)^2 - 1450246047))];
%  
%                                                                                                         (43164*sin(theta_1 + theta_2)*(7700*cos(theta_2) + 6329))/(3388000*cos(theta_2)^2 - 1450246047) - (759480000000*u)/(7*(3388000*cos(theta_2)^2 - 1450246047)) - theta_d_2*((160*(7700*cos(theta_2) + 6329))/(7*(3388000*cos(theta_2)^2 - 1450246047)) + (50632000000*sin(theta_2)*((77*theta_d_1)/200000 + (77*theta_d_2)/200000))/(7*(3388000*cos(theta_2)^2 - 1450246047))) - (50632000000*((75537*sin(theta_1 + theta_2))/2000000 + (38259*sin(theta_1))/800000))/(7*(3388000*cos(theta_2)^2 - 1450246047)) - theta_d_1*((50632000000*((77*theta_d_2*sin(theta_2))/200000 - 5171/250))/(7*(3388000*cos(theta_2)^2 - 1450246047)) + (440*theta_d_1*sin(theta_2)*(7700*cos(theta_2) + 6329))/(3388000*cos(theta_2)^2 - 1450246047))
% theta_d_2*((80*(30800*cos(theta_2) + 8032663))/(7*(3388000*cos(theta_2)^2 - 1450246047)) + (8000000*sin(theta_2)*((77*theta_d_1)/200000 + (77*theta_d_2)/200000)*(7700*cos(theta_2) + 6329))/(7*(3388000*cos(theta_2)^2 - 1450246047))) + theta_d_1*((8000000*((77*theta_d_2*sin(theta_2))/200000 - 5171/250)*(7700*cos(theta_2) + 6329))/(7*(3388000*cos(theta_2)^2 - 1450246047)) + (220*theta_d_1*sin(theta_2)*(30800*cos(theta_2) + 8032663))/(3388000*cos(theta_2)^2 - 1450246047)) + (120000000*u*(7700*cos(theta_2) + 6329))/(7*(3388000*cos(theta_2)^2 - 1450246047)) - (21582*sin(theta_1 + theta_2)*(30800*cos(theta_2) + 8032663))/(3388000*cos(theta_2)^2 - 1450246047) + (8000000*(7700*cos(theta_2) + 6329)*((75537*sin(theta_1 + theta_2))/2000000 + (38259*sin(theta_1))/800000))/(7*(3388000*cos(theta_2)^2 - 1450246047))
%  

% T_d_new = (T - T_prev)/1;


theta_dd_val = [
                                                                                                                                                                   (2177205792337185200000*sin(theta_1 + theta_2)*(7101996468378179*cos(theta_2) + 5837472162125388))/(59390441777463697512*cos(theta_2) + 157619855740175396464645510487628125*cos(theta_2)^2 - 67469767625708245300871903596602750000) - theta_d_2*((1152921504606846976*(7101996468378179*cos(theta_2) + 5837472162125388))/(59390441777463697512*cos(theta_2) + 157619855740175396464645510487628125*cos(theta_2)^2 - 67469767625708245300871903596602750000) + (336507359412909324930676272031334400000*sin(theta_2)*((7101996468378179*theta_d_1)/18446744073709551616 + (7101996468378179*theta_d_2)/18446744073709551616))/(59390441777463697512*cos(theta_2) + 157619855740175396464645510487628125*cos(theta_2)^2 - 67469767625708245300871903596602750000)) - theta_d_1*((336507359412909324930676272031334400000*((7101996468378179*theta_d_2*sin(theta_2))/18446744073709551616 - 5171/250))/(59390441777463697512*cos(theta_2) + 157619855740175396464645510487628125*cos(theta_2)^2 - 67469767625708245300871903596602750000) + (22193738963681809375*theta_d_1*sin(theta_2)*(7101996468378179*cos(theta_2) + 5837472162125388))/(59390441777463697512*cos(theta_2) + 157619855740175396464645510487628125*cos(theta_2)^2 - 67469767625708245300871903596602750000)) - (336507359412909324930676272031334400000*T)/(59390441777463697512*cos(theta_2) + 157619855740175396464645510487628125*cos(theta_2)^2 - 67469767625708245300871903596602750000) - (336507359412909324930676272031334400000*((5443014480842963*sin(theta_1 + theta_2))/144115188075855872 + (3446064362871357*sin(theta_1))/72057594037927936))/(59390441777463697512*cos(theta_2) + 157619855740175396464645510487628125*cos(theta_2)^2 - 67469767625708245300871903596602750000);
theta_d_1*((57646075230342348800000*(7101996468378179*cos(theta_2) + 5837472162125388)*((7101996468378179*theta_d_2*sin(theta_2))/18446744073709551616 - 5171/250))/(59390441777463697512*cos(theta_2) + 157619855740175396464645510487628125*cos(theta_2)^2 - 67469767625708245300871903596602750000) + (7272444383619255296*theta_d_1*sin(theta_2)*(43347146413441024*cos(theta_2) + 11304968154247740625))/(59390441777463697512*cos(theta_2) + 157619855740175396464645510487628125*cos(theta_2)^2 - 67469767625708245300871903596602750000)) + theta_d_2*((1180591620717411303424*(43347146413441024*cos(theta_2) + 11304968154247740625))/(3125*(59390441777463697512*cos(theta_2) + 157619855740175396464645510487628125*cos(theta_2)^2 - 67469767625708245300871903596602750000)) + (57646075230342348800000*sin(theta_2)*(7101996468378179*cos(theta_2) + 5837472162125388)*((7101996468378179*theta_d_1)/18446744073709551616 + (7101996468378179*theta_d_2)/18446744073709551616))/(59390441777463697512*cos(theta_2) + 157619855740175396464645510487628125*cos(theta_2)^2 - 67469767625708245300871903596602750000)) + (57646075230342348800000*T*(7101996468378179*cos(theta_2) + 5837472162125388))/(59390441777463697512*cos(theta_2) + 157619855740175396464645510487628125*cos(theta_2)^2 - 67469767625708245300871903596602750000) + (57646075230342348800000*(7101996468378179*cos(theta_2) + 5837472162125388)*((5443014480842963*sin(theta_1 + theta_2))/144115188075855872 + (3446064362871357*sin(theta_1))/72057594037927936))/(59390441777463697512*cos(theta_2) + 157619855740175396464645510487628125*cos(theta_2)^2 - 67469767625708245300871903596602750000) - (713426794033048846336*sin(theta_1 + theta_2)*(43347146413441024*cos(theta_2) + 11304968154247740625))/(59390441777463697512*cos(theta_2) + 157619855740175396464645510487628125*cos(theta_2)^2 - 67469767625708245300871903596602750000)     
];

== matlab function pole_placement_oldversion/Subsystem2/set_limit_rad ==
  settings: updateMethod=DISCRETE  sampleTime=0.001
  data: theta_old input size=1; theta_new output size=1
function theta_new   = set_limit_rad(theta_old)

theta_new = theta_old - floor(theta_old / 2 / pi) * 2 * pi;
theta_new = theta_old;

== matlab function pole_placement_oldversion/Subsystem2/set_limit_rad1 ==
  settings: updateMethod=DISCRETE  sampleTime=0.001
  data: theta_old input size=1; theta_new output size=1
function theta_new   = set_limit_rad(theta_old)

theta_new = theta_old - floor(theta_old / 2 / pi) * 2 * pi;
theta_new = theta_old;

== matlab function pole_placement_oldversion/Subsystem2/set_limit_rad2 ==
  settings: updateMethod=DISCRETE  sampleTime=0.001
  data: theta_old input size=1; theta_new output size=1
function theta_new   = set_limit_rad(theta_old)

theta_new = theta_old - floor(theta_old / 2 / pi) * 2 * pi;
theta_new = theta_old;

== matlab function pole_placement_oldversion/Subsystem2/set_limit_rad3 ==
  settings: updateMethod=DISCRETE  sampleTime=0.001
  data: theta_old input size=1; theta_new output size=1
function theta_new   = set_limit_rad(theta_old)

theta_new = theta_old - floor(theta_old / 2 / pi) * 2 * pi;
theta_new = theta_old;

== matlab function pole_placement_oldversion/Subsystem2/set_limit_rad4 ==
  settings: updateMethod=DISCRETE  sampleTime=0.001
  data: theta_old input size=1; theta_new output size=1
function theta_new   = set_limit_rad(theta_old)

theta_new = theta_old - floor(theta_old / 2 / pi) * 2 * pi;
theta_new = theta_old;

== matlab function pole_placement_oldversion/Subsystem2/set_limit_rad5 ==
  settings: updateMethod=DISCRETE  sampleTime=0.001
  data: theta_old input size=1; theta_new output size=1
function theta_new   = set_limit_rad(theta_old)

theta_new = theta_old - floor(theta_old / 2 / pi) * 2 * pi;
theta_new = theta_old;
